simulink model "IK_rate_controller_PWM_Control_Mode 3"  (R2025b)
settings: Solver=FixedStepAuto  StartTime=0.0  StopTime=14  FixedStep=Ts  RelTol=1e-3
undefined symbols (not defined in the file or in its folder): motor_IDs, Ts
libraries: dspindex x5, dspsigops x4, simulink_extras x3, dxlSimLibrary x3, robotcorelib x1, sldrtlib x1
settings Model: Creator=ziyad  LastModifiedBy=ziyad
settings SolverCC: EnableFixedStepZeroCrossing=on
settings OptimizationCC: DefaultParameterBehavior=Inlined  EnhancedBackFolding=on  PassReuseOutputArgsThreshold=0.0  MaxStackSize=200000  OptimizeBlockOrder=speed  DifferentSizesBufferReuse=on
settings DebuggingCC: ParameterTunabilityLossMsg=error
settings HardwareCC: ProdBitPerLong=64.0  ProdHWDeviceType=Intel->x86-64 (Linux 64)
settings SFSimCC: MATLABDynamicMemAlloc=off
settings RTWCC: SystemTargetFile=sldrt.tlc  TemplateMakefile=sldrt.tmf  RTWCompilerOptimization=on  Description=Simulink Desktop Real-Time
settings CodeAppCC: ForceParamTrailComments=on  MaxIdLength=95.0  OperatorAnnotations=on
settings SimulinkDesktopRealTimeCC: ExtModeTransport=0.0  ExtModeStaticAllocSize=1000000.0  TargetLibSuffix=_sldrt.a  TargetPreCompLibLocation=C:\Program Files\MATLAB\R2025b\toolbox\sldrt\lib\win64  TargetLangStandard=C89/C90 (ANSI)  MultiwordLength=2048.0  DynamicStringBufferSize=256.0  ParMdlRefBuildCompliant=on  PreserveMATLABNamespacesInGeneratedCode=on  SubcomponentCodeInterfacePackaging=Reusable function

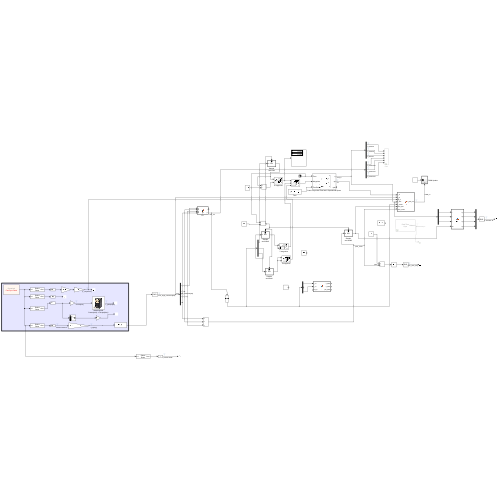
[thumbnail: Simulink's stored preview of the top-level diagram]
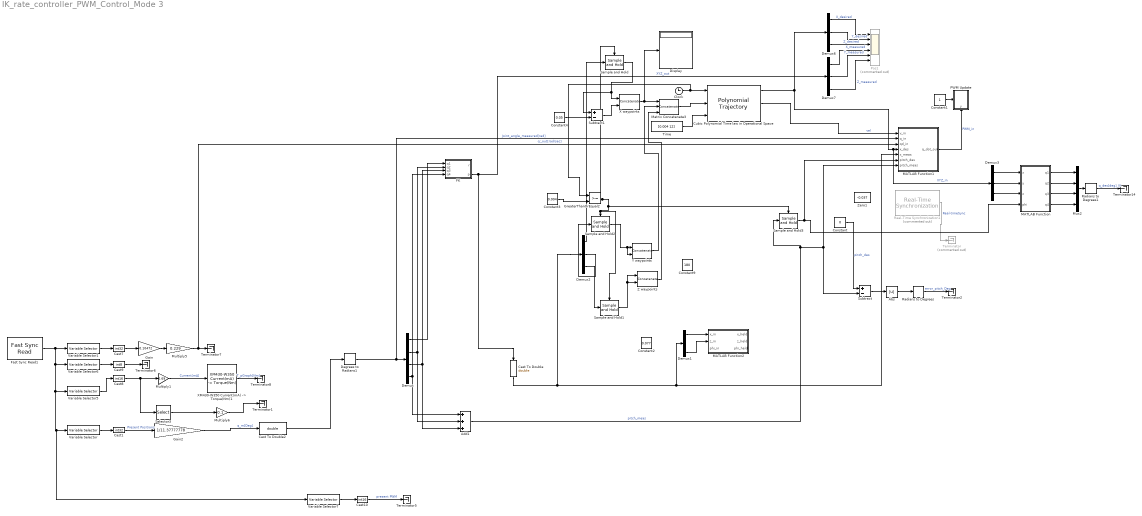
== system IK_rate_controller_PWM_Control_Mode 3 ==
  Abs : Abs  SaturateOnIntegerOverflow=off
  Add1 : Sum  Inputs=+++
  Cast To Double : DataTypeConversion  OutDataTypeStr=double  SaturateOnIntegerOverflow=off  RndMeth=Floor
  Cast To Double2 : DataTypeConversion  OutDataTypeStr=double  SaturateOnIntegerOverflow=off  RndMeth=Floor
  Cast1 : DataTypeConversion  OutDataTypeStr=int32  SaturateOnIntegerOverflow=off  RndMeth=Floor
  Cast10 : DataTypeConversion  OutDataTypeStr=int16  SaturateOnIntegerOverflow=off  RndMeth=Floor
  Cast7 : DataTypeConversion  OutDataTypeStr=int32  SaturateOnIntegerOverflow=off  RndMeth=Floor
  Cast8 : DataTypeConversion  OutDataTypeStr=int16  SaturateOnIntegerOverflow=off  RndMeth=Floor
  Cast9 : DataTypeConversion  OutDataTypeStr=int8  SaturateOnIntegerOverflow=off  RndMeth=Floor
  Clock : Clock
  Constant : Constant  Value=0
  Constant1 : Constant
  Constant2 : Constant  Value=0.077
  Constant3 : Constant  Value=0.004
  Constant4 : Constant  Value=0.05
  Constant9 : Constant  Value=180
  Cubic Polynomial Time law in Operational Space : robotcorelib/Polynomial Trajectory  WaypointSource=External  Waypoints=[0.25,0.25,0.15; 0,0,0; 0.1 ,0.1,0.1]  TimePoints=[1,2,3]  TimeInterval=[ 2, 20 ]  Method=Quintic Polynomial  ParameterSource=Internal  VelocityBoundaryCondition=zeros(3,2)  AccelerationBoundaryCondition=zeros( 3,2 )  SimulateUsing=Interpreted execution
  Degrees to Radians1 : simulink_extras/Transformations/Degrees to Radians
  Demux : Demux
  Demux{1..3,6..7} (5 alike) : Demux  Outputs=3
  Display : Display
  FK : MATLAB Function  TreatAsAtomicUnit=on
  Fast Sync Read1 : dxlSimLibrary/Fast Sync Read  lib_name='dxl_x64_c'  group_num_read=group_num_read  ids=motor_IDs  models=motor_models  select_sync_read=select_sync_read  start_address_read_indirect=start_address_read_indirect  Ts=Ts
  Gain : Gain  Gain=0.10472
  Gain2 : Gain  Gain=1/11.37777778
  GreaterThanOrEqual2 : RelationalOperator  OutDataTypeStr=boolean  RndMeth=Simplest  InputSameDT=off
  MATLAB Function : MATLAB Function  TreatAsAtomicUnit=on
  MATLAB Function1 : MATLAB Function  TreatAsAtomicUnit=on
  MATLAB Function2 : MATLAB Function  TreatAsAtomicUnit=on
  Matrix Concatenate3 : Concatenate  NumInputs=3  Mode=Multidimensional array
  Multiply1 : Gain  Gain=2.69  OutDataTypeStr=double
  Multiply5 : Gain  Gain=0.229  OutDataTypeStr=double
  Multiply6 : Gain  Gain=0.1  OutDataTypeStr=double
  Mux2 : Mux
  PWM Update : Subsystem  TreatAsAtomicUnit=on
  Pos1 : Scope  Commented=on  NumInputPorts=6
      settings: Title=Time history with a cubic polynomial time law  ActiveDisplayYMinimum=-0.034681761003191973  ActiveDisplayYMaximum=0.29962437658108865  YLabel=Position [m]  DataLoggingVariableName=ScopeData9
  Radians to Degrees : simulink_extras/Transformations/Radians to Degrees
  Radians to Degrees1 : simulink_extras/Transformations/Radians to Degrees
  Real-Time Synchronization1 : sldrtlib/Real-Time Synchronization  Commented=on  SampleTime=Ts  MaxMissedTicks=10000  ShowMissedTicks=on  YieldWhenWaiting=off
  Sample and Hold : dspsigops/Sample and Hold  trig=Rising edge  initCond=0.233  latchinput=off
  Sample and Hold1 : dspsigops/Sample and Hold  trig=Rising edge  initCond=0.026  latchinput=off
  Sample and Hold2 : dspsigops/Sample and Hold  trig=Rising edge  initCond=0  latchinput=off
  Sample and Hold3 : dspsigops/Sample and Hold  trig=Rising edge  initCond=0  latchinput=off
  Selector3 : Selector  InputPortWidth=length(motor_IDs)  IndexOptions=Index vector (dialog)  Indices=1  OutputSizes=1
  Subtract : Sum  Inputs=+-
  Subtract1 : Sum  Inputs=+-
  Terminator : Terminator  Commented=on
  Terminator{1..2,5..8,14} (7 alike) : Terminator
  Time : Constant  Value=[0.004 12]
  Variable Selector : dspindex/Variable Selector  NumInputs=1  rowsOrCols=Rows  IdxMode=Fixed  Elements=1  ZerOneIdxMode=One-based  errmode=Clip Index  FillMode=on  FillValues=0
  Variable Selector1 : dspindex/Variable Selector  NumInputs=1  rowsOrCols=Rows  IdxMode=Fixed  Elements=2  ZerOneIdxMode=One-based  errmode=Clip Index  FillMode=on  FillValues=0
  Variable Selector5 : dspindex/Variable Selector  NumInputs=1  rowsOrCols=Rows  IdxMode=Fixed  Elements=3  ZerOneIdxMode=One-based  errmode=Clip Index  FillMode=on  FillValues=0
  Variable Selector6 : dspindex/Variable Selector  NumInputs=1  rowsOrCols=Rows  IdxMode=Fixed  Elements=4  ZerOneIdxMode=One-based  errmode=Clip Index  FillMode=on  FillValues=0
  Variable Selector7 : dspindex/Variable Selector  NumInputs=1  rowsOrCols=Rows  IdxMode=Fixed  Elements=5  ZerOneIdxMode=One-based  errmode=Clip Index  FillMode=on  FillValues=0
  X waypoints : Concatenate  Mode=Multidimensional array  ConcatenateDimension=2
  "XM430-W350 Current(mA) -> Torque(Nm)1" : dxlSimLibrary/Subsystem/XM430-W350 /XM430-W350 Current(mA) -> Torque(Nm)  SystemSampleTime=-1  VariantActivationTime=update diagram  EmptyChoice=off  PassThrough=off  PassThroughVariantControl=(default)  EmptyChoiceVariantControl=(default)  AllowFlexibleInterface=on  Latency=0  AutoFrameSizeCalculation=off
  Y waypoints : Concatenate  Mode=Multidimensional array  ConcatenateDimension=2
  Z waypoints : Concatenate  Mode=Multidimensional array  ConcatenateDimension=2
  Zero1 : Constant  Value=-0.037  OutDataTypeStr=Inherit: Inherit via back propagation
  wires:
  Clock/1 -> GreaterThanOrEqual2/1, Cubic Polynomial Time law in Operational Space/1
  Demux2/3 -> Sample and Hold1/1
  Demux2/2 -> Sample and Hold2/1
  Real-Time Synchronization1/1 -> Terminator/1  "Real-timeSync"
  Constant1/1 -> PWM Update/Enable
  Time/1 -> Cubic Polynomial Time law in Operational Space/3
  Degrees to Radians1/1 -> MATLAB Function1/2(q_in), Demux/1  "Joint_angle_measured[rad]"
  Demux/2 -> Add1/2, FK/2(q2)
  Demux/1 -> FK/1(q1)
  Demux/4 -> FK/4(q4), Add1/1
  Demux/3 -> FK/3(q3), Add1/3
  FK/2(p) -> Demux7/1, Cast To Double/1  "XYZ_out"
  Add1/1 -> Sample and Hold3/1, Subtract/2, MATLAB Function1/7(pitch_meas)  "pitch_meas"
  Cast To Double/1 -> MATLAB Function1/5(x_meas), Demux1/1, Demux2/1
  Matrix Concatenate3/1 -> Cubic Polynomial Time law in Operational Space/2
  X waypoints/1 -> Display/1, Matrix Concatenate3/1
  Y waypoints/1 -> Matrix Concatenate3/2
  Demux6/3 -> Pos1/3  "Z_desired"
  Demux6/2 -> Pos1/2  "Y_desired"
  Demux6/1 -> Pos1/1  "X_desired"
  Z waypoints/1 -> Matrix Concatenate3/3
  Cubic Polynomial Time law in Operational Space/2 -> MATLAB Function1/1(v_in)  "vel"
  Cubic Polynomial Time law in Operational Space/1 -> Demux3/1, MATLAB Function1/4(x_des), Demux6/1  "XYZ_in"
  Demux7/3 -> Pos1/6  "Z_measured"
  Demux7/2 -> Pos1/5  "Y_measured"
  Demux7/1 -> Pos1/4  "X_measured"
  "XM430-W350 Current(mA) -> Torque(Nm)1"/1 -> Terminator8/1  "T_pGraph[Nm]"
  Variable Selector5/1 -> Cast8/1
  Multiply6/1 -> Terminator1/1
  Cast9/1 -> Terminator6/1
  Variable Selector1/1 -> Cast7/1
  Selector3/1 -> Multiply6/1
  Cast To Double2/1 -> Degrees to Radians1/1
  Variable Selector/1 -> Cast1/1
  Cast8/1 -> Selector3/1, Multiply1/1
  Cast7/1 -> Gain/1
  Cast1/1 -> Gain2/1  "Present Positions"
  Gain2/1 -> Cast To Double2/1  "q_m[Deg]"
  Multiply5/1 -> MATLAB Function1/3(qd_in), Terminator7/1  "q'_out[rad/sec]"
  Variable Selector6/1 -> Cast9/1
  Multiply1/1 -> "XM430-W350 Current(mA) -> Torque(Nm)1"/1  "Current[mA]"
  Gain/1 -> Multiply5/1
  Constant/1 -> Subtract/1  "pitch_des"
  MATLAB Function1/1(q_dot_out) -> PWM Update/1(y)  "PWM_in"
  Subtract/1 -> Abs/1
  Abs/1 -> Radians to Degrees/1
  Radians to Degrees/1 -> Terminator2/1  "error_pitch_Deg"
  Variable Selector7/1 -> Cast10/1
  Fast Sync Read1/1 -> Variable Selector7/1, Variable Selector/1, Variable Selector5/1, Variable Selector6/1, Variable Selector1/1
  Cast10/1 -> Terminator5/1  "present PWM"
  Demux1/1 -> MATLAB Function2/1(x_in)
  Demux1/3 -> MATLAB Function2/2(z_in)
  Demux3/1 -> MATLAB Function/1(x)
  Demux3/2 -> MATLAB Function/2(y)
  Demux3/3 -> MATLAB Function/3(z)
  MATLAB Function/1(q1) -> Mux2/1
  MATLAB Function/2(q2) -> Mux2/2
  MATLAB Function/3(q3) -> Mux2/3
  MATLAB Function/4(q4) -> Mux2/4
  Mux2/1 -> Radians to Degrees1/1
  Radians to Degrees1/1 -> Terminator14/1  "q_des[deg]_IK"
  Sample and Hold/1 -> Subtract1/1, X waypoints/1
  Subtract1/1 -> X waypoints/2
  Constant4/1 -> Subtract1/2
  Sample and Hold1/1 -> Z waypoints/2, Z waypoints/1
  Constant3/1 -> GreaterThanOrEqual2/2
  GreaterThanOrEqual2/1 -> Sample and Hold3/Trigger, Sample and Hold1/Trigger, Sample and Hold2/Trigger, Sample and Hold/Trigger
  Sample and Hold2/1 -> Y waypoints/2, Y waypoints/1
  Demux2/1 -> Sample and Hold/1
  Sample and Hold3/1 -> MATLAB Function1/6(pitch_des), MATLAB Function/4(phi)

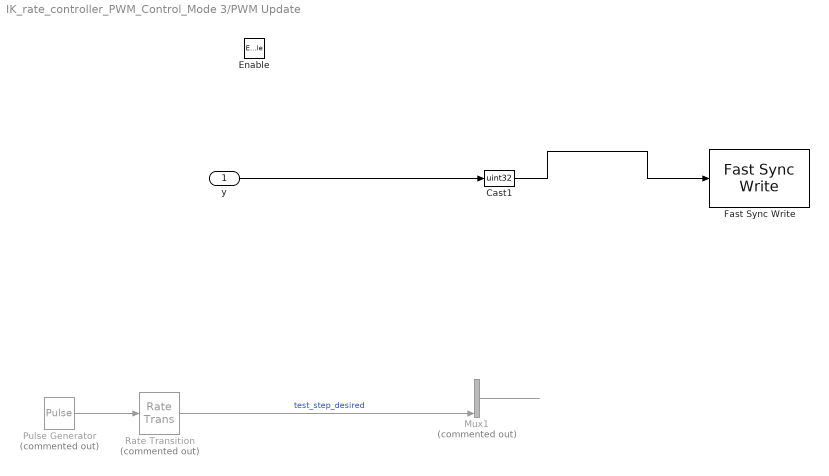
== system IK_rate_controller_PWM_Control_Mode 3/PWM Update ==
  y : Inport
  Enable : EnablePort
  Cast1 : DataTypeConversion  OutMin=0  OutMax=2097150  OutDataTypeStr=uint32  SaturateOnIntegerOverflow=off  RndMeth=Floor
  Fast Sync Write : dxlSimLibrary/Fast Sync Write  Description=|  lib_name=lib_name  group_num_write=group_num_write  ids=motor_IDs  models=motor_models  select_sync_write=select_sync_write  Ts=Ts
      | Dynamixel library for Matlab and Simulink
      | Fast Sync Write function
      | Author: Georgios Andrikopoulos (geoand@kth.se), 2022 
      | Mechatronics & Embedded Control Systems Unit, KTH, Stockholm
  Mux1 : Mux  Commented=on
  Pulse Generator : DiscretePulseGenerator  Commented=on  PulseType=Time based  Amplitude=15  Period=1  PulseWidth=50  PhaseDelay=0.5
  Rate Transition : RateTransition  Commented=on  OutPortSampleTime=Ts
  wires:
  y/1 -> Cast1/1
  Cast1/1 -> Fast Sync Write/1
  Mux1/1 -> ?
  Pulse Generator/1 -> Rate Transition/1
  Rate Transition/1 -> Mux1/4  "test_step_desired"

== matlab function IK_rate_controller_PWM_Control_Mode 3/MATLAB Function ==
  data: x input; q1 output; y input; z input; phi input; q2 output; q3 output; q4 output
function [q1,q2,q3,q4] = fcn(x,y,z,phi)
    % Link parameters
    a2 = 0.13; a3 = 0.124; a4 = 0.0815;
    d1 = 0.077;

    % Base angle
    q1 = atan2(y,x);

    % Wrist center position sqrt(x^2 + z^2)
    pwx = sqrt(x^2 + y^2) - a4*cos(phi);
    pwz = z - d1 - a4*sin(phi);

    % Distance from shoulder to wrist center
    dist = sqrt(pwx^2 + pwz^2);

    %Reachability check
    if dist > (a2 + a3) || dist < abs(a2 - a3)
        error('Target point is outside the reachable workspace');
    end

    % Compute q3
    c3 = (pwx^2 + pwz^2 - a2^2 - a3^2)/(2*a2*a3);
    s3 = -sqrt(1 - c3^2); % (-)elbow-up (use +s3 for elbow-down)
    q3 = atan2(s3,c3);
% beta = atan2(a3*s3, a2 + a3*c3)
% gamma = atan2(pwz,pwx)
    % Compute q2
    q2 = atan2(pwz,pwx) - atan2(a3*s3, a2 + a3*c3)
    % Compute q4
    q4 = phi - (q2 + q3);
   
end

== matlab function IK_rate_controller_PWM_Control_Mode 3/MATLAB Function1 ==
  data: v_in input; q_dot_out output; q_in input; qd_in input; x_des input; x_meas input; pitch_des input; pitch_meas input
function q_dot_out = fcn(v_in, q_in, qd_in, x_des, x_meas, pitch_des, pitch_meas)
v_in       = double(v_in);
q_in       = double(q_in);
qd_in      = double(qd_in(:));
x_des      = double(x_des);
x_meas     = double(x_meas);
pitch_des  = double(pitch_des);
pitch_meas = double(pitch_meas);

Ts = 1/500;
l1 = 0.130;
l2 = 0.124;
l3 = 0.0815;

q_dot_lim = 600.0;

persistent int_x_err int_pitch_err
if isempty(int_x_err)
    int_x_err     = zeros(3,1);
    int_pitch_err = 0;
end

q1 = q_in(1);
q2 = q_in(2);
q3 = q_in(3);
q4 = q_in(4);

s1   = sin(q1);   c1   = cos(q1);
s2   = sin(q2);   c2   = cos(q2);
s23  = sin(q2+q3); c23  = cos(q2+q3);
s234 = sin(q2+q3+q4); c234 = cos(q2+q3+q4);

R = l1*c2 + l2*c23 + l3*c234;
J = zeros(3,4);
J(:,1) = [-s1*R; c1*R; 0];
J(:,2) = [-c1*(l1*s2 + l2*s23 + l3*s234);
          -s1*(l1*s2 + l2*s23 + l3*s234);
           l1*c2 + l2*c23 + l3*c234];
J(:,3) = [-c1*(l2*s23 + l3*s234);
          -s1*(l2*s23 + l3*s234);
           l2*c23 + l3*c234];
J(:,4) = [-c1*l3*s234; -s1*l3*s234; l3*c234];

J_o = [0 1 1 1];
J_aug = [J; J_o];

JJt = J_aug * J_aug';
mu  = sqrt(max(det(JJt), 0));
mu_thresh   = 0.01;
lambda_min  = 1e-3;
lambda_max  = 5e-2;
if mu < mu_thresh
    lambda = lambda_max * (1 - (mu/mu_thresh)^2);
else
    lambda = lambda_min;
end
J_pinv = J_aug' / (JJt + lambda^2*eye(4));

x_err     = x_des     - x_meas;
pitch_err = pitch_des - pitch_meas;

v_meas    = J_aug * qd_in;
v_err_lin = v_in - v_meas(1:3);
omega_err = -v_meas(4);

% Kp_x     = diag([1800, 1700, 2500]);
% Kd_x     = diag([  20,   20,   30]);
% Ki_x     = diag([ 285,  285,  300]);

Kp_x     = diag([4.3250,    4.3250,    9.7311]*10^3); %diag([50, 50, 50]*1.5*1.5*1.5*1.5*1.5*1.5*1.5*1.5*1.5*1.5);
Kd_x     = diag([  0,   0,   0]);
Ki_x     = diag([ 20,  20,  20]);

Kp_pitch =  3.4172*10^3*1.5;%200*1.5*1.5*1.5*1.5*1.5*1.5*1.5;
Kd_pitch = 0;
Ki_pitch = 10;

v_lin_cmd = v_in ...
            + Kp_x  * x_err ...
            + Kd_x  * v_err_lin ...
            + Ki_x  * int_x_err;
omega_cmd =   Kp_pitch * pitch_err ...
            + Kd_pitch * omega_err ...
            + Ki_pitch * int_pitch_err;

z_bias = 22;
v_lin_cmd(3) = v_lin_cmd(3) + z_bias;

v_cmd = [v_lin_cmd; omega_cmd];

q_dot_unsat = J_pinv * v_cmd;
q_dot_out = max(min(q_dot_unsat, q_dot_lim), -q_dot_lim);

%q_dot_out = q_dot_unsat;

int_x_err     = int_x_err     + x_err     * Ts;
int_pitch_err = int_pitch_err + pitch_err * Ts;

int_x_err     = max(min(int_x_err,     0.02), -0.02);
int_pitch_err = max(min(int_pitch_err, 0.2 ), -0.2 );

end

== matlab function IK_rate_controller_PWM_Control_Mode 3/FK ==
  data: q1 input; r output; q2 input; q3 input; q4 input; p output
function [r,p] = fcn(q1,q2,q3,q4)

% D-H parameters. 
a1 = 0;     alpha1 = 1/2;  d1 = 0.077;
a2 = 0.13;  alpha2 = 0;     d2 = 0;
a3 = 0.124; alpha3 = 0;     d3 = 0;
a4 = 0.0815; alpha4 = 0;     d4 = 0;

T = @(theta, d, a, alpha) [cos(theta), -sin(theta)*cospi(alpha),  sin(theta)*sinpi(alpha), a*cos(theta);
                           sin(theta),  cos(theta)*cospi(alpha), -cos(theta)*sinpi(alpha), a*sin(theta);
                           0,           sinpi(alpha),             cospi(alpha),            d;
                           0,           0,                      0,                     1];

T1 = T(q1, d1, a1, alpha1);
T2 = T(q2, d2, a2, alpha2);
T3 = T(q3, d3, a3, alpha3);
T4 = T(q4, d4, a4, alpha4);


T = T1*T2*T3*T4;
r = T(1:3,1:3);
p = T(1:3,4);

== matlab function IK_rate_controller_PWM_Control_Mode 3/MATLAB Function2 ==
  data: x_in input; x_held output; z_in input; phi_in input; z_held output; phi_held output
function [x_held, z_held, phi_held] = fcn(x_in, z_in, phi_in)
%#codegen
persistent x0 z0 phi0 captured
if isempty(captured)
    x0       = x_in;
    z0       = z_in;
    phi0     = phi_in;
    captured = true;
end
x_held   = x0;
z_held   = z0;
phi_held = phi0;
end
